simulink model "Solution1"  (R2024b)
settings: Solver=VariableStepAuto  StartTime=0.0  StopTime=10.0  RelTol=1e-3
settings Model: Creator=saibot  LastModifiedBy=saibot

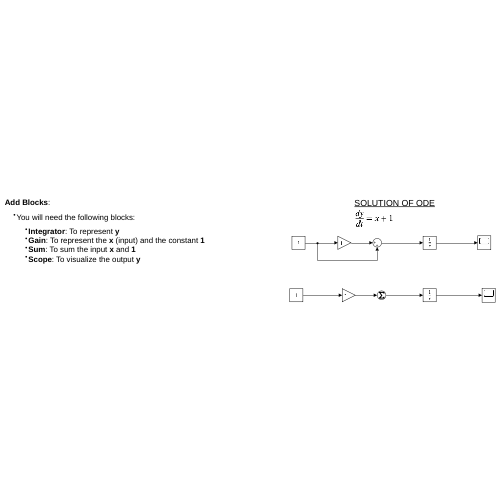
[thumbnail: Simulink's stored preview of the top-level diagram]
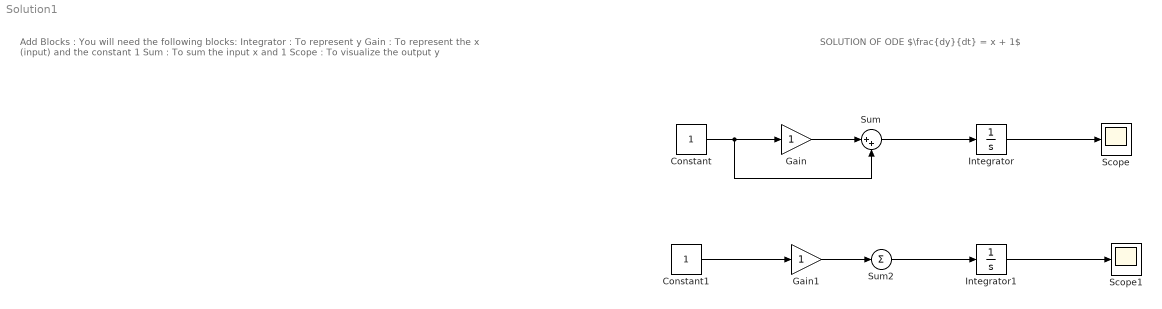
== system Solution1 ==
  note: Add Blocks :
      | You will need the following blocks: Integrator : To represent y
      | Gain : To represent the x (input) and the constant 1
      | Sum : To sum the input x and 1
      | Scope : To visualize the output y
  note: SOLUTION OF ODE
      | $\frac{dy}{dt} = x + 1$
  Constant : Constant
  Constant1 : Constant
  Gain : Gain
  Gain1 : Gain
  Integrator : Integrator
  Integrator1 : Integrator
  Scope : Scope
  Scope1 : Scope
  Sum : Sum  Inputs=|++
  Sum2 : Sum  Inputs=|+|
  wires:
  Sum/1 -> Integrator/1
  Integrator/1 -> Scope/1
  Constant/1 -> Sum/2, Gain/1
  Gain/1 -> Sum/1
  Constant1/1 -> Gain1/1
  Gain1/1 -> Sum2/1
  Sum2/1 -> Integrator1/1
  Integrator1/1 -> Scope1/1
